simulink model "closedmodi"  (R2020a)
settings: Solver=VariableStepAuto  StartTime=0.0  StopTime=1  RelTol=1e-3
libraries: powerlib x38, simulink x1, simulink_extras x1
settings Model: Creator=Ratish Kumar S  LastModifiedBy=Ratish Kumar S
settings DataIOCC: ReturnWorkspaceOutputs=off
settings DebuggingCC: ArithmeticOperatorsInVariantConditions=warning
settings SFSimCC: CustomCodeUndefinedFunction=UseInterfaceOnly

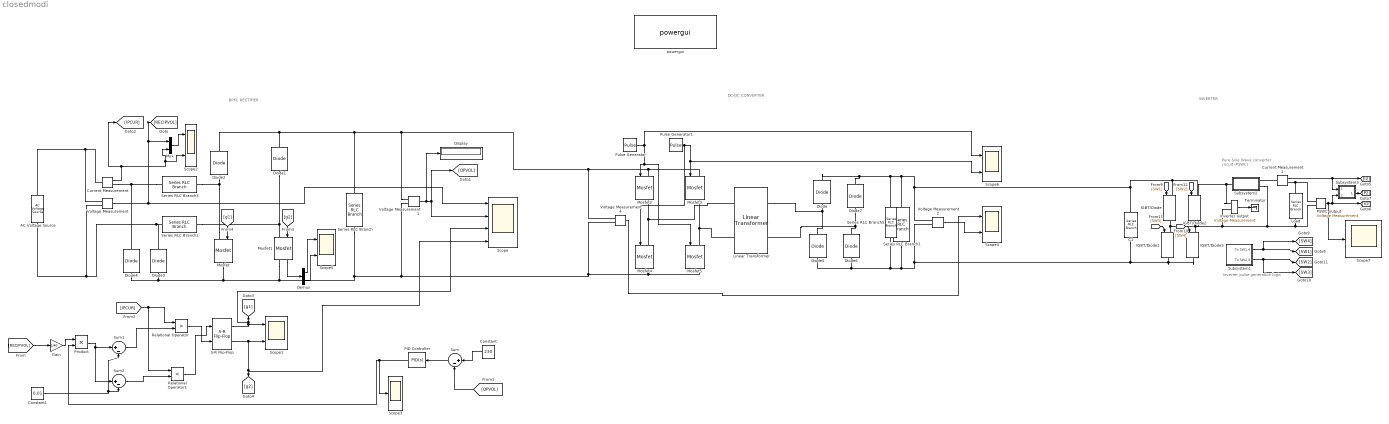
== system closedmodi ==
  note: INVERTER
  note: DC-DC CONVERTER
  note: Inverter pulse generation logic
  note: BPFC RECTIFIER
  note: Pure Sine Wave converter circuit (PSWC)
  AC Voltage Source : powerlib/Electrical Sources/AC Voltage Source  Amplitude=230  Phase=0  Frequency=50  SampleTime=0  Measurements=None  BusType=swing  Pref=10e3  Qref=0  Qmin=-inf  Qmax=+inf
  C1 : powerlib/Elements/Series RLC Branch  LConnTagsString=__new0  RConnTagsString=__new0  BranchType=C  Resistance=1  Inductance=1e-3  SetiL0=off  InitialCurrent=0  Capacitance=200e-3  Setx0=off  InitialVoltage=0  Measurements=None
  Constant : Constant  Value=230
  Constant1 : Constant  Value=0.01
  Current Measurement : powerlib/Measurements/Current Measurement  PhasorSimulation=off  OutputType=Complex  PSBequivalent=0
  Current Measurement1 : powerlib/Measurements/Current Measurement  PhasorSimulation=off  OutputType=Complex  PSBequivalent=0
  Demux : Demux  Outputs=2
  Diode{,1..7} (8 alike) : powerlib/Power Electronics/Diode  Ron=0.001  Lon=0  Vf=0.8  IC=0  UseSnubber=off  Rs=500  Cs=250e-9  Measurements=off
  Display : Display
  Gain : Gain  Gain=1/40
  IGBT/Diode{,1..3} (4 alike) : powerlib/Power Electronics/IGBT//Diode  Ron=1e-3  Rs=1e5  Cs=inf  Measurements=off
  Inverter output : powerlib/Measurements/Voltage Measurement  PhasorSimulation=off  OutputType=Complex  PSBequivalent=0
  Linear Transformer : powerlib/Elements/Linear Transformer  UNITS=SI  NominalPower=[5e3 50000 ]  winding1=[300 0.0004 0]  winding2=[170 0.0004 0]  ThreeWindings=off  winding3=[3.15e+05 24806 7.8961]  RmLm=[1000 21.518e-6]  Measurements=None  DataType=on
  Load : powerlib/Elements/Series RLC Branch  LConnTagsString=__new0  RConnTagsString=__new0  BranchType=R  Resistance=8  Inductance=10e-3  SetiL0=off  InitialCurrent=0  Capacitance=100e-6  Setx0=off  InitialVoltage=0  Measurements=None
  Mosfet : powerlib/Power Electronics/Mosfet  Ron=0.1  Lon=0  Rd=0.01  Vfd=0  IC=0  Rs=1e5  Cs=inf  Measurements=off
  Mosfet1 : powerlib/Power Electronics/Mosfet  Ron=0.1  Lon=0  Rd=0.01  Vfd=0  IC=0  Rs=1e5  Cs=inf  Measurements=on
  Mosfet{2..5} (4 alike) : powerlib/Power Electronics/Mosfet  Ron=2e-3  Lon=0  Rd=2e-3  Vfd=1  IC=0  Rs=1e5  Cs=inf  Measurements=on
  Mux : Mux  Inputs=2
  PID Controller : simulink/Continuous/PID Controller  Controller=PID  Form=Parallel  TimeDomain=Continuous-time  UseExternalTs=off  SampleTime=-1  IntegratorMethod=Forward Euler  FilterMethod=Forward Euler  ControllerParametersSource=internal  P=-0.01  I=1  D=7.5  UseFilter=on  N=1  TunerSelectOption=Transfer Function Based (PID Tuner App)  ZeroCross=off  InitialConditionSource=internal  InitialConditionForIntegrator=0  InitialConditionForFilter=0  DifferentiatorICPrevScaledInput=0  ExternalReset=none  TrackingMode=off  Kt=1  LimitOutput=off  UpperSaturationLimit=inf  LowerSaturationLimit=-inf  LinearizeAsGain=on  AntiWindupMode=none  Kb=1  POutMin=[]  POutMax=[]  IOutMin=[]  IOutMax=[]  DOutMin=[]  DOutMax=[]  NOutMin=[]  NOutMax=[]  SumOutMin=[]  SumOutMax=[]  SaturationOutMin=[]  SaturationOutMax=[]  PParamMin=[]  PParamMax=[]  IParamMin=[]  IParamMax=[]  DParamMin=[]  DParamMax=[]  NParamMin=[]  NParamMax=[]  KbParamMin=[]  KbParamMax=[]  KtParamMin=[]  KtParamMax=[]  KbOutMin=[]  KbOutMax=[]  KtOutMin=[]  KtOutMax=[]  IntegratorOutMin=[]  IntegratorOutMax=[]  FilterOutMin=[]  FilterOutMax=[]  SumI1OutMin=[]  SumI1OutMax=[]  SumI2OutMin=[]  SumI2OutMax=[]  SumI3OutMin=[]  SumI3OutMax=[]  SumI4OutMin=[]  SumI4OutMax=[]  SumDOutMin=[]  SumDOutMax=[]  DifferentiatorOutMin=[]  DifferentiatorOutMax=[]  FilterDiffOutCoefMin=[]  FilterDiffOutCoefMax=[]  ReciprocalOutMin=[]  ReciprocalOutMax=[]  SumDenOutMin=[]  SumDenOutMax=[]  SumNumOutMin=[]  SumNumOutMax=[]  DivideOutMin=[]  DivideOutMax=[]  UdiffTsProdOutMin=[]  UdiffTsProdOutMax=[]  NTsProdOutMin=[]  NTsProdOutMax=[]  UintegralTsProdOutMin=[]  UintegralTsProdOutMax=[]  UngainTsProdOutMin=[]  UngainTsProdOutMax=[]  IntegratorContinuousStateAttributes=''  IntegratorStateMustResolveToSignalObject=off  IntegratorRTWStateStorageClass=Auto  FilterContinuousStateAttributes=''  FilterStateMustResolveToSignalObject=off  FilterRTWStateStorageClass=Auto  ParallelPVariant=InternalParameters  IdealPVariant=Disabled  IVariant=InternalParameters  DVariant=InternalParameters  IntegratorVariant=Continuous  SatVariant=Disabled  AWVariant=Passthrough  PCopyVariant=Disabled  TRVariant=Disabled  FdbkBlocksVariant=Forward  IdealPFdbkVariant=Disabled  SatFdbkVariant=Disabled  DerivativeFilterVariant=ContFilter  NVariant=InternalParameters  NCopyVariant=Disabled  FilterICVariant=InternalICsFilter  IntegratorICVariant=InternalICs  ExternalResetVariant=Disabled  TRSumVariant=Passthrough  SumFdbkVariant=Disabled  SumVariant=Sum_PID  TsampFilterVariant=InternalTs  TsampNgainVariant=Passthrough  TsampIntegralVariant=Passthrough
  PSWC output : powerlib/Measurements/Voltage Measurement  PhasorSimulation=off  OutputType=Complex  PSBequivalent=0
  Product : Product
  Pulse Generator : DiscretePulseGenerator  PulseType=Time based  Period=.00002  PulseWidth=50  VectorParams1D=off
  Pulse Generator1 : DiscretePulseGenerator  PulseType=Time based  Period=.00002  PulseWidth=50  PhaseDelay=2.22e-10  VectorParams1D=off
  Relational Operator : RelationalOperator  Operator=>  OutDataTypeStr=boolean  RndMeth=Nearest
  Relational Operator1 : RelationalOperator  Operator=<  OutDataTypeStr=boolean  RndMeth=Nearest
  S-R Flip-Flop : simulink_extras/Flip Flops/S-R Flip-Flop  initial_condition=0
  Scope : Scope  NumInputPorts=4
  Scope{1..2,4..6} (5 alike) : Scope  NumInputPorts=2
  Scope3 : Scope
  Scope7 : Scope
  Series RLC Branch : powerlib/Elements/Series RLC Branch  LConnTagsString=__new0  RConnTagsString=__new0  BranchType=C  Resistance=1  Inductance=1e-3  SetiL0=off  InitialCurrent=0  Capacitance=100e-6  Setx0=off  InitialVoltage=0  Measurements=None
  Series RLC Branch1 : powerlib/Elements/Series RLC Branch  LConnTagsString=__new0  RConnTagsString=__new0  BranchType=R  Resistance=100  Inductance=1e-3  SetiL0=off  InitialCurrent=0  Capacitance=1e-6  Setx0=off  InitialVoltage=0  Measurements=None
  Series RLC Branch2 : powerlib/Elements/Series RLC Branch  LConnTagsString=__new0  RConnTagsString=__new0  BranchType=L  Resistance=1  Inductance=5e-3  SetiL0=off  InitialCurrent=0  Capacitance=1e-6  Setx0=off  InitialVoltage=0  Measurements=None
  Series RLC Branch3 : powerlib/Elements/Series RLC Branch  LConnTagsString=__new0  RConnTagsString=__new0  BranchType=L  Resistance=1  Inductance=5e-3  SetiL0=off  InitialCurrent=0  Capacitance=1e-6  Setx0=off  InitialVoltage=0  Measurements=None
  Series RLC Branch5 : powerlib/Elements/Series RLC Branch  LConnTagsString=__new0  RConnTagsString=__new0  BranchType=C  Resistance=1  Inductance=1e-3  SetiL0=off  InitialCurrent=0  Capacitance=300e-5  Setx0=off  InitialVoltage=0  Measurements=Branch voltage
  Subsystem1 : Subsystem
  Subsystem2 : Subsystem
  Subsystem3 : Subsystem
  Sum : Sum  Inputs=|+-
  Sum1 : Sum  Inputs=|+-
  Sum2 : Sum  Inputs=|+-
  Terminator : Terminator
  Voltage Measurement{,1..2,4} (4 alike) : powerlib/Measurements/Voltage Measurement  PhasorSimulation=off  OutputType=Complex  PSBequivalent=0
  powergui : powerlib/powergui  Priority=1  SimulationMode=Discrete  SampleTime=1e-6  frequency=60  Iterations=50  frequencyindice=0  Pbase=100e6  ErrMax=1e-4  UnitsV=kV  UnitsW=MW  buscounter=0  FunctionMessages=off  echomessages=off  EnableUseOfTLC=off  CurrentSourceSwitches=off  DisableSnubberDevices=off  DisableRonSwitches=off  DisableVfSwitches=off  DisplayEquations=off  AutomaticDiscreteSolvers=off  SolverType=Tustin/Backward Euler (TBE)  Interpol=off  ExternalGateDelay=off  methode=off  Ts=100  x0status=blocks  SPID=off  SwTol=0  HookPort=off  NonlinearTolerance=1e-4  nMaxIteration=100  ContinueOnMaxIteration=off  RestoreLinks=warning  ResistiveCurrentMeasurement=off  Frange=[0:2:500]  Ylog=off  Xlog=on  ShowGrid=off  save=off  variable=ZData  structure=0  ZoomFFT=off  StartTime=0.0  cycles=1  DisplayStyle=1  fundamental=60  FreqAxis=off  MaxFrequency=1000  frequencyindicesteady=1  RmsSteady=1  display=off
  wires:
  Current Measurement1/1 -> Subsystem3/1(In1), [I2]
  Subsystem3/1(Out1) -> [P2]
  Subsystem1/2(To SW2,3) -> [SW3], [SW2]
  [SW1] -> IGBT/Diode/1
  [SW4] -> IGBT/Diode3/1
  [SW2] -> IGBT/Diode2/1
  Inverter output/1 -> Terminator/1
  [SW3] -> IGBT/Diode1/1
  Mux/1 -> Scope2/1
  S-R Flip-Flop/2 -> [g2], Scope/4, Scope1/2
  Pulse Generator1/1 -> Scope6/2, Mosfet3/1, Mosfet4/1
  PSWC output/1 -> Scope7/1, [V2], Subsystem3/2(In2)
  Pulse Generator/1 -> Scope6/1, Mosfet2/1, Mosfet5/1
  Voltage Measurement4/1 -> Scope4/1
  Relational Operator/1 -> S-R Flip-Flop/2
  [OPVOL] -> Sum/2
  Voltage Measurement1/1 -> Display/1, [OPVOL], Scope/2
  Constant1/1 -> Sum1/2, Sum2/2
  PID Controller/1 -> Scope3/1, Product/2
  Voltage Measurement2/1 -> Scope4/2
  Relational Operator1/1 -> S-R Flip-Flop/1
  [g2] -> Mosfet1/1
  Sum2/1 -> Relational Operator1/2
  Sum1/1 -> Relational Operator/2
  [IPCUR] -> Relational Operator1/1, Relational Operator/1
  Subsystem1/1(To SW1,4) -> [SW1], [SW4]
  Voltage Measurement/1 -> Scope/1, [RECIPVOL], Mux/1
  [RECIPVOL] -> Gain/1
  Gain/1 -> Product/1
  S-R Flip-Flop/1 -> Scope/3, [g1], Scope1/1
  Current Measurement/1 -> Scope2/2, Mux/2, [IPCUR]
  Constant/1 -> Sum/1
  Sum/1 -> PID Controller/1
  [g1] -> Mosfet/1
  Product/1 -> Sum2/1, Sum1/1
  Mosfet1/1 -> Demux/1
  Demux/1 -> Scope5/1
  Demux/2 -> Scope5/2
  connections:
  Current Measurement1/RConn1 -- Load/LConn1 -- PSWC output/LConn1
  IGBT/Diode2/RConn1 -- IGBT/Diode3/LConn1 -- Inverter output/LConn2 -- Subsystem2/RConn2 -- Load/RConn1 -- PSWC output/LConn2
  Inverter output/LConn1 -- Subsystem2/LConn1 -- IGBT/Diode1/LConn1 -- IGBT/Diode/RConn1
  Diode5/LConn1 -- Diode6/LConn1 -- Series RLC Branch5/RConn1 -- Voltage Measurement2/LConn2 -- C1/RConn1 -- IGBT/Diode3/RConn1 -- IGBT/Diode1/RConn1 -- Series RLC Branch1/RConn1
  Diode5/RConn1 -- Linear Transformer/RConn1 -- Diode/LConn1
  Diode7/RConn1 -- Series RLC Branch5/LConn1 -- IGBT/Diode/LConn1 -- IGBT/Diode2/LConn1 -- C1/LConn1 -- Voltage Measurement2/LConn1 -- Series RLC Branch1/LConn1 -- Diode/RConn1
  Mosfet1/RConn1 -- Series RLC Branch/RConn1 -- Mosfet5/RConn1 -- Mosfet4/RConn1 -- Voltage Measurement4/LConn2 -- Voltage Measurement1/LConn2 -- Diode3/LConn1 -- Diode4/LConn1 -- Mosfet/RConn1
  Mosfet3/RConn1 -- Linear Transformer/LConn2 -- Mosfet5/LConn1
  Linear Transformer/RConn2 -- Diode6/RConn1 -- Diode7/LConn1
  Mosfet/LConn1 -- Diode2/LConn1 -- Series RLC Branch3/RConn1
  Voltage Measurement1/LConn1 -- Voltage Measurement4/LConn1 -- Mosfet3/LConn1 -- Mosfet2/LConn1 -- Series RLC Branch/LConn1 -- Diode2/RConn1 -- Diode1/RConn1
  Mosfet2/RConn1 -- Linear Transformer/LConn1 -- Mosfet4/LConn1
  AC Voltage Source/LConn1 -- Voltage Measurement/LConn2 -- Diode3/RConn1 -- Series RLC Branch2/LConn1
  Series RLC Branch3/LConn1 -- Diode4/RConn1 -- Current Measurement/RConn1
  AC Voltage Source/RConn1 -- Voltage Measurement/LConn1 -- Current Measurement/LConn1
  Mosfet1/LConn1 -- Series RLC Branch2/RConn1 -- Diode1/LConn1
  Current Measurement1/LConn1 -- Subsystem2/RConn1

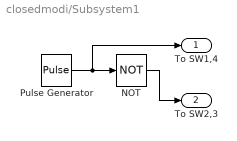
== system closedmodi/Subsystem1 ==
  NOT : Logic  Operator=NOT  IconShape=distinctive  AllPortsSameDT=off  OutDataTypeStr=boolean
  Pulse Generator : DiscretePulseGenerator  PulseType=Time based  Period=1/50  PulseWidth=50
  To SW1,4 : Outport  VectorParamsAs1DForOutWhenUnconnected=off
  To SW2,3 : Outport  Port=2  VectorParamsAs1DForOutWhenUnconnected=off
  wires:
  NOT/1 -> To SW2,3/1
  Pulse Generator/1 -> To SW1,4/1, NOT/1

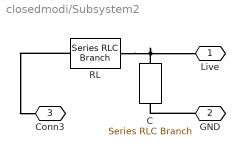
== system closedmodi/Subsystem2 ==
  C : powerlib/Elements/Series RLC Branch  LConnTagsString=__new0  RConnTagsString=__new0  BranchType=C  Resistance=1  Inductance=1e-3  SetiL0=off  InitialCurrent=0  Capacitance=300e-6  Setx0=off  InitialVoltage=0  Measurements=None
  RL : powerlib/Elements/Series RLC Branch  LConnTagsString=__new0  RConnTagsString=__new0  BranchType=RL  Resistance=1.25  Inductance=40e-3  SetiL0=off  InitialCurrent=0  Capacitance=1000e-6  Setx0=off  InitialVoltage=0  Measurements=None
  Live : PMIOPort  Side=Right
  GND : PMIOPort  Port=2  Side=Right
  Conn3 : PMIOPort  Port=3  Side=Left
  connections:
  GND/RConn1 -- C/RConn1
  RL/LConn1 -- Conn3/RConn1
  C/LConn1 -- Live/RConn1 -- RL/RConn1

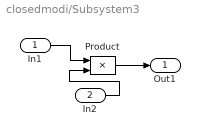
== system closedmodi/Subsystem3 ==
  In1 : Inport
  In2 : Inport  Port=2
  Product : Product
  Out1 : Outport  VectorParamsAs1DForOutWhenUnconnected=off
  wires:
  In2/1 -> Product/2
  In1/1 -> Product/1
  Product/1 -> Out1/1
